simulink model "add_waves"  (R2020a)
settings: Solver=VariableStepAuto  StartTime=0.0  StopTime=10.0  MaxStep=.001  RelTol=1e-3
libraries: simulink x1
settings Model: Creator=Administrator  LastModifiedBy=Administrator

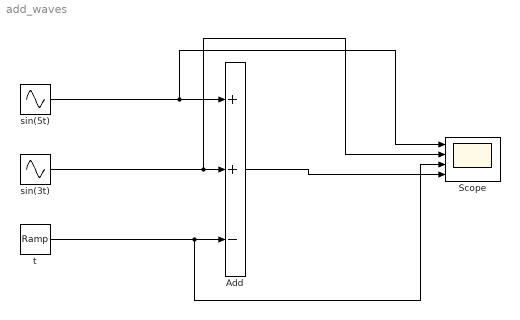
== system add_waves ==
  Add : Sum  Inputs=++-
  Scope : Scope  NumInputPorts=4
  sin(3t) : Sin  Frequency=2*3*pi  SampleTime=0
  sin(5t) : Sin  Frequency=2*5*pi  SampleTime=0
  t : simulink/Sources/Ramp  slope=1  start=0  InitialOutput=0
  wires:
  sin(5t)/1 -> Scope/1, Add/1
  sin(3t)/1 -> Scope/2, Add/2
  t/1 -> Scope/3, Add/3
  Add/1 -> Scope/4
